simulink library "INT_HPUn_Co"  (R2016b)
settings: Solver=VariableStepAuto  StartTime=0.0  StopTime=10.0  RelTol=1e-3
settings Model: Creator=lenovo  LastModifiedBy=lenovo

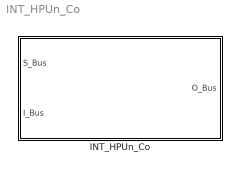
== system INT_HPUn_Co ==
  INT_HPUn_Co : Subsystem

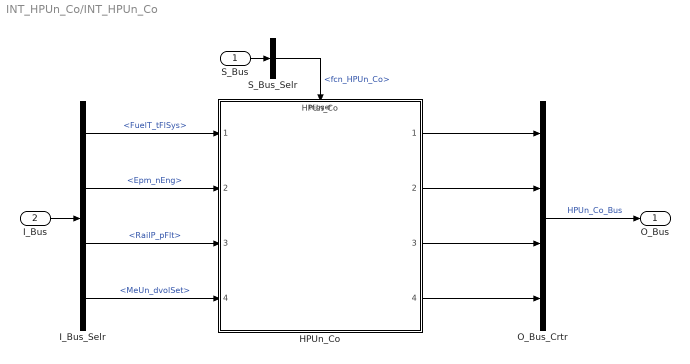
== system INT_HPUn_Co/INT_HPUn_Co ==
  S_Bus : Inport
  I_Bus : Inport  Port=2
  HPUn_Co : ModelReference  ModelNameDialog=HPUn_Co  SimulationMode=Normal  ModelReferenceVersion=1.20  TriggerPortName=function  TriggerPortTriggerType=function-call  TriggerPortStatesWhenEnabling=held
  I_Bus_Selr : BusSelector  OutputSignals=FuelT_tFlSys,Epm_nEng,RailP_pFlt,MeUn_dvolSet
  O_Bus_Crtr : BusCreator  Inputs=4
  S_Bus_Selr : BusSelector  OutputSignals=fcn_HPUn_Co
  O_Bus : Outport
  wires:
  S_Bus_Selr/1 -> HPUn_Co/Trigger  "<fcn_HPUn_Co>"
  S_Bus/1 -> S_Bus_Selr/1
  I_Bus/1 -> I_Bus_Selr/1
  I_Bus_Selr/1 -> HPUn_Co/1  "<FuelT_tFlSys>"
  I_Bus_Selr/2 -> HPUn_Co/2  "<Epm_nEng>"
  I_Bus_Selr/3 -> HPUn_Co/3  "<RailP_pFlt>"
  I_Bus_Selr/4 -> HPUn_Co/4  "<MeUn_dvolSet>"
  O_Bus_Crtr/1 -> O_Bus/1  "HPUn_Co_Bus"
  HPUn_Co/1 -> O_Bus_Crtr/1
  HPUn_Co/2 -> O_Bus_Crtr/2
  HPUn_Co/3 -> O_Bus_Crtr/3
  HPUn_Co/4 -> O_Bus_Crtr/4
